simulink model "pv_array2"  (R2015a)
settings: Solver=ode45  StartTime=0.0  StopTime=10  RelTol=1e-3
undefined symbols (not defined in the file or in its folder): sigbuilder_block
libraries: powerlib x24
(part 2 of 2)

== system pv_array2/PV_array /PV module6/PV module/Photon Curr  ==
  "Tak " : Inport
  Trk : Inport  Port=2
  Isc,ref : Inport  Port=3
  "Insolation " : Inport  Port=4
  Ki : Inport  Port=5
  " " : Constant  Value=1000
  Divide : Product  Inputs=*/
  Product : Product
  Product1 : Product
  Sum1 : Sum  Inputs=|++
  Sum2 : Sum  Inputs=|+-
  "Iph " : Outport
  wires:
  "Tak "/1 -> Sum2/1
  Trk/1 -> Sum2/2
  Sum2/1 -> Product/2
  Product/1 -> Sum1/1
  Isc,ref/1 -> Sum1/2
  "Insolation "/1 -> Divide/1
  " "/1 -> Divide/2
  Divide/1 -> Product1/1
  Product1/1 -> "Iph "/1
  Sum1/1 -> Product1/2
  Ki/1 -> Product/1

== system pv_array2/PV_array /PV module6/PV module/Reverse Sat Cur  ==
  "Tak " : Inport
  "Isc ref " : Inport  Port=2
  q : Inport  Port=3
  Voc : Inport  Port=4
  k : Inport  Port=5
  "A " : Inport  Port=6
  "Constant " : Constant
  Divide : Product  Inputs=**////
  Fcn : Fcn  Expr=u(1)/(exp(u(2))-u(3))
  Mux : Mux  Inputs=3
  "Ns " : Constant  Value=36
  Irs : Outport
  wires:
  "Tak "/1 -> Divide/6
  "Ns "/1 -> Divide/4
  "Isc ref "/1 -> Mux/1
  Divide/1 -> Mux/2
  "Constant "/1 -> Mux/3
  Mux/1 -> Fcn/1
  Fcn/1 -> Irs/1
  q/1 -> Divide/1
  Voc/1 -> Divide/2
  k/1 -> Divide/3
  "A "/1 -> Divide/5

== system pv_array2/PV_array /PV module6/PV module/Sat Curr ==
  Irs : Inport
  Tak : Inport  Port=2
  Trk : Inport  Port=3
  q : Inport  Port=4
  Eg0 : Inport  Port=5
  k : Inport  Port=6
  B : Inport  Port=7
  " " : Constant
  Divide : Product  Inputs=*/
  Divide1 : Product  Inputs=***//
  Divide2 : Product  Inputs=*/
  Divide3 : Product  Inputs=*/
  Fcn : Fcn  Expr=(u(1))^3
  Math Function : Math  SaturateOnIntegerOverflow=on
  Product1 : Product  Inputs=3
  Sum : Sum  Inputs=|+-
  Is : Outport
  wires:
  Sum/1 -> Divide1/3
  Fcn/1 -> Product1/2
  Divide/1 -> Fcn/1
  Product1/1 -> Is/1
  Math Function/1 -> Product1/1
  Divide1/1 -> Math Function/1
  Tak/1 -> Divide3/2, Divide/1
  Irs/1 -> Product1/3
  " "/1 -> Divide3/1, Divide2/1
  Trk/1 -> Divide2/2, Divide/2
  Divide2/1 -> Sum/1
  Divide3/1 -> Sum/2
  q/1 -> Divide1/1
  Eg0/1 -> Divide1/2
  k/1 -> Divide1/4
  B/1 -> Divide1/5

== system pv_array2/PV_array /PV module7/PV module/Cel to Kel ==
  "Top " : Inport
  Add : Sum
  Add1 : Sum
  Cel to Kel : Constant  Value=273
  T(ref ^C)1 : Constant  Value=25
  "Tak " : Outport
  "Trk " : Outport  Port=2
  wires:
  Add/1 -> "Tak "/1
  Add1/1 -> "Trk "/1
  T(ref ^C)1/1 -> Add1/1
  Cel to Kel/1 -> Add1/2, Add/2
  "Top "/1 -> Add/1

== system pv_array2/PV_array /PV module7/PV module/NsAkt ==
  TaK : Inport
  Ns : Inport  Port=2
  k : Inport  Port=3
  A : Inport  Port=4
  Product : Product  Inputs=4
  Naskt : Outport
  wires:
  Product/1 -> Naskt/1
  TaK/1 -> Product/4
  Ns/1 -> Product/1
  k/1 -> Product/2
  A/1 -> Product/3

== system pv_array2/PV_array /PV module7/PV module/PV-Panel Current ==
  Is : Inport
  "Vpv " : Inport  Port=2
  NsAkT : Inport  Port=3
  "Iph " : Inport  Port=4
  Np : Inport  Port=5
  q : Inport  Port=6
  Fcn : Fcn  Expr=u(7)*u(2)-u(6)*u(2)*(exp((u(3)*(u(4)+u(5))/u(1)))-1)
  Mux : Mux  Inputs=7
  Rs : Gain  Gain=0.45
  Ipv : Outport
  wires:
  NsAkT/1 -> Mux/1
  Fcn/1 -> Ipv/1, Rs/1
  Rs/1 -> Mux/5
  "Iph "/1 -> Mux/7
  Is/1 -> Mux/6
  "Vpv "/1 -> Mux/4
  Mux/1 -> Fcn/1
  Np/1 -> Mux/2
  q/1 -> Mux/3

== system pv_array2/PV_array /PV module7/PV module/Photon Curr  ==
  "Tak " : Inport
  Trk : Inport  Port=2
  Isc,ref : Inport  Port=3
  "Insolation " : Inport  Port=4
  Ki : Inport  Port=5
  " " : Constant  Value=1000
  Divide : Product  Inputs=*/
  Product : Product
  Product1 : Product
  Sum1 : Sum  Inputs=|++
  Sum2 : Sum  Inputs=|+-
  "Iph " : Outport
  wires:
  "Tak "/1 -> Sum2/1
  Trk/1 -> Sum2/2
  Sum2/1 -> Product/2
  Product/1 -> Sum1/1
  Isc,ref/1 -> Sum1/2
  "Insolation "/1 -> Divide/1
  " "/1 -> Divide/2
  Divide/1 -> Product1/1
  Product1/1 -> "Iph "/1
  Sum1/1 -> Product1/2
  Ki/1 -> Product/1

== system pv_array2/PV_array /PV module7/PV module/Reverse Sat Cur  ==
  "Tak " : Inport
  "Isc ref " : Inport  Port=2
  q : Inport  Port=3
  Voc : Inport  Port=4
  k : Inport  Port=5
  "A " : Inport  Port=6
  "Constant " : Constant
  Divide : Product  Inputs=**////
  Fcn : Fcn  Expr=u(1)/(exp(u(2))-u(3))
  Mux : Mux  Inputs=3
  "Ns " : Constant  Value=36
  Irs : Outport
  wires:
  "Tak "/1 -> Divide/6
  "Ns "/1 -> Divide/4
  "Isc ref "/1 -> Mux/1
  Divide/1 -> Mux/2
  "Constant "/1 -> Mux/3
  Mux/1 -> Fcn/1
  Fcn/1 -> Irs/1
  q/1 -> Divide/1
  Voc/1 -> Divide/2
  k/1 -> Divide/3
  "A "/1 -> Divide/5

== system pv_array2/PV_array /PV module7/PV module/Sat Curr ==
  Irs : Inport
  Tak : Inport  Port=2
  Trk : Inport  Port=3
  q : Inport  Port=4
  Eg0 : Inport  Port=5
  k : Inport  Port=6
  B : Inport  Port=7
  " " : Constant
  Divide : Product  Inputs=*/
  Divide1 : Product  Inputs=***//
  Divide2 : Product  Inputs=*/
  Divide3 : Product  Inputs=*/
  Fcn : Fcn  Expr=(u(1))^3
  Math Function : Math  SaturateOnIntegerOverflow=on
  Product1 : Product  Inputs=3
  Sum : Sum  Inputs=|+-
  Is : Outport
  wires:
  Sum/1 -> Divide1/3
  Fcn/1 -> Product1/2
  Divide/1 -> Fcn/1
  Product1/1 -> Is/1
  Math Function/1 -> Product1/1
  Divide1/1 -> Math Function/1
  Tak/1 -> Divide3/2, Divide/1
  Irs/1 -> Product1/3
  " "/1 -> Divide3/1, Divide2/1
  Trk/1 -> Divide2/2, Divide/2
  Divide2/1 -> Sum/1
  Divide3/1 -> Sum/2
  q/1 -> Divide1/1
  Eg0/1 -> Divide1/2
  k/1 -> Divide1/4
  B/1 -> Divide1/5

== system pv_array2/PV_array /PV module8/PV module/Cel to Kel ==
  "Top " : Inport
  Add : Sum
  Add1 : Sum
  Cel to Kel : Constant  Value=273
  T(ref ^C)1 : Constant  Value=25
  "Tak " : Outport
  "Trk " : Outport  Port=2
  wires:
  Add/1 -> "Tak "/1
  Add1/1 -> "Trk "/1
  T(ref ^C)1/1 -> Add1/1
  Cel to Kel/1 -> Add1/2, Add/2
  "Top "/1 -> Add/1

== system pv_array2/PV_array /PV module8/PV module/NsAkt ==
  TaK : Inport
  Ns : Inport  Port=2
  k : Inport  Port=3
  A : Inport  Port=4
  Product : Product  Inputs=4
  Naskt : Outport
  wires:
  Product/1 -> Naskt/1
  TaK/1 -> Product/4
  Ns/1 -> Product/1
  k/1 -> Product/2
  A/1 -> Product/3

== system pv_array2/PV_array /PV module8/PV module/PV-Panel Current ==
  Is : Inport
  "Vpv " : Inport  Port=2
  NsAkT : Inport  Port=3
  "Iph " : Inport  Port=4
  Np : Inport  Port=5
  q : Inport  Port=6
  Fcn : Fcn  Expr=u(7)*u(2)-u(6)*u(2)*(exp((u(3)*(u(4)+u(5))/u(1)))-1)
  Mux : Mux  Inputs=7
  Rs : Gain  Gain=0.45
  Ipv : Outport
  wires:
  NsAkT/1 -> Mux/1
  Fcn/1 -> Ipv/1, Rs/1
  Rs/1 -> Mux/5
  "Iph "/1 -> Mux/7
  Is/1 -> Mux/6
  "Vpv "/1 -> Mux/4
  Mux/1 -> Fcn/1
  Np/1 -> Mux/2
  q/1 -> Mux/3

== system pv_array2/PV_array /PV module8/PV module/Photon Curr  ==
  "Tak " : Inport
  Trk : Inport  Port=2
  Isc,ref : Inport  Port=3
  "Insolation " : Inport  Port=4
  Ki : Inport  Port=5
  " " : Constant  Value=1000
  Divide : Product  Inputs=*/
  Product : Product
  Product1 : Product
  Sum1 : Sum  Inputs=|++
  Sum2 : Sum  Inputs=|+-
  "Iph " : Outport
  wires:
  "Tak "/1 -> Sum2/1
  Trk/1 -> Sum2/2
  Sum2/1 -> Product/2
  Product/1 -> Sum1/1
  Isc,ref/1 -> Sum1/2
  "Insolation "/1 -> Divide/1
  " "/1 -> Divide/2
  Divide/1 -> Product1/1
  Product1/1 -> "Iph "/1
  Sum1/1 -> Product1/2
  Ki/1 -> Product/1

== system pv_array2/PV_array /PV module8/PV module/Reverse Sat Cur  ==
  "Tak " : Inport
  "Isc ref " : Inport  Port=2
  q : Inport  Port=3
  Voc : Inport  Port=4
  k : Inport  Port=5
  "A " : Inport  Port=6
  "Constant " : Constant
  Divide : Product  Inputs=**////
  Fcn : Fcn  Expr=u(1)/(exp(u(2))-u(3))
  Mux : Mux  Inputs=3
  "Ns " : Constant  Value=36
  Irs : Outport
  wires:
  "Tak "/1 -> Divide/6
  "Ns "/1 -> Divide/4
  "Isc ref "/1 -> Mux/1
  Divide/1 -> Mux/2
  "Constant "/1 -> Mux/3
  Mux/1 -> Fcn/1
  Fcn/1 -> Irs/1
  q/1 -> Divide/1
  Voc/1 -> Divide/2
  k/1 -> Divide/3
  "A "/1 -> Divide/5

== system pv_array2/PV_array /PV module8/PV module/Sat Curr ==
  Irs : Inport
  Tak : Inport  Port=2
  Trk : Inport  Port=3
  q : Inport  Port=4
  Eg0 : Inport  Port=5
  k : Inport  Port=6
  B : Inport  Port=7
  " " : Constant
  Divide : Product  Inputs=*/
  Divide1 : Product  Inputs=***//
  Divide2 : Product  Inputs=*/
  Divide3 : Product  Inputs=*/
  Fcn : Fcn  Expr=(u(1))^3
  Math Function : Math  SaturateOnIntegerOverflow=on
  Product1 : Product  Inputs=3
  Sum : Sum  Inputs=|+-
  Is : Outport
  wires:
  Sum/1 -> Divide1/3
  Fcn/1 -> Product1/2
  Divide/1 -> Fcn/1
  Product1/1 -> Is/1
  Math Function/1 -> Product1/1
  Divide1/1 -> Math Function/1
  Tak/1 -> Divide3/2, Divide/1
  Irs/1 -> Product1/3
  " "/1 -> Divide3/1, Divide2/1
  Trk/1 -> Divide2/2, Divide/2
  Divide2/1 -> Sum/1
  Divide3/1 -> Sum/2
  q/1 -> Divide1/1
  Eg0/1 -> Divide1/2
  k/1 -> Divide1/4
  B/1 -> Divide1/5

== system pv_array2/PV_array /PV module9/PV module/Cel to Kel ==
  "Top " : Inport
  Add : Sum
  Add1 : Sum
  Cel to Kel : Constant  Value=273
  T(ref ^C)1 : Constant  Value=25
  "Tak " : Outport
  "Trk " : Outport  Port=2
  wires:
  Add/1 -> "Tak "/1
  Add1/1 -> "Trk "/1
  T(ref ^C)1/1 -> Add1/1
  Cel to Kel/1 -> Add1/2, Add/2
  "Top "/1 -> Add/1

== system pv_array2/PV_array /PV module9/PV module/NsAkt ==
  TaK : Inport
  Ns : Inport  Port=2
  k : Inport  Port=3
  A : Inport  Port=4
  Product : Product  Inputs=4
  Naskt : Outport
  wires:
  Product/1 -> Naskt/1
  TaK/1 -> Product/4
  Ns/1 -> Product/1
  k/1 -> Product/2
  A/1 -> Product/3

== system pv_array2/PV_array /PV module9/PV module/PV-Panel Current ==
  NsAkT : Inport
  Np : Inport  Port=2
  q : Inport  Port=3
  "Vpv " : Inport  Port=4
  Is : Inport  Port=5
  "Iph " : Inport  Port=6
  Display : Display
  Display1 : Display
  Display2 : Display
  Fcn : Fcn  Expr=u(7)*u(2)-u(6)*u(2)*(exp((u(3)*(u(4)+u(5))/u(1)))-1)
  Mux : Mux  Inputs=7
  Rs : Gain  Gain=0.45
  Ipv : Outport
  wires:
  NsAkT/1 -> Mux/1
  Fcn/1 -> Ipv/1, Display2/1, Rs/1
  "Iph "/1 -> Mux/6, Display/1
  Is/1 -> Mux/5, Display1/1
  "Vpv "/1 -> Mux/4
  Mux/1 -> Fcn/1
  Np/1 -> Mux/2
  q/1 -> Mux/3
  Rs/1 -> Mux/7

== system pv_array2/PV_array /PV module9/PV module/Photon Curr  ==
  "Tak " : Inport
  Trk : Inport  Port=2
  Isc,ref : Inport  Port=3
  "Insolation " : Inport  Port=4
  Ki : Inport  Port=5
  " " : Constant  Value=1000
  Divide : Product  Inputs=*/
  Product : Product
  Product1 : Product
  Sum1 : Sum  Inputs=|++
  Sum2 : Sum  Inputs=|+-
  "Iph " : Outport
  wires:
  "Tak "/1 -> Sum2/1
  Trk/1 -> Sum2/2
  Sum2/1 -> Product/2
  Product/1 -> Sum1/1
  Isc,ref/1 -> Sum1/2
  "Insolation "/1 -> Divide/1
  " "/1 -> Divide/2
  Divide/1 -> Product1/1
  Product1/1 -> "Iph "/1
  Sum1/1 -> Product1/2
  Ki/1 -> Product/1

== system pv_array2/PV_array /PV module9/PV module/Reverse Sat Cur  ==
  "Tak " : Inport
  "Isc ref " : Inport  Port=2
  q : Inport  Port=3
  Voc : Inport  Port=4
  k : Inport  Port=5
  "A " : Inport  Port=6
  "Constant " : Constant
  Divide : Product  Inputs=**////
  Fcn : Fcn  Expr=u(1)/(exp(u(2))-u(3))
  Mux : Mux  Inputs=3
  "Ns " : Constant  Value=36
  Irs : Outport
  wires:
  "Tak "/1 -> Divide/6
  "Ns "/1 -> Divide/4
  "Isc ref "/1 -> Mux/1
  Divide/1 -> Mux/2
  "Constant "/1 -> Mux/3
  Mux/1 -> Fcn/1
  Fcn/1 -> Irs/1
  q/1 -> Divide/1
  Voc/1 -> Divide/2
  k/1 -> Divide/3
  "A "/1 -> Divide/5

== system pv_array2/PV_array /PV module9/PV module/Sat Curr ==
  Irs : Inport
  Tak : Inport  Port=2
  Trk : Inport  Port=3
  q : Inport  Port=4
  Eg0 : Inport  Port=5
  k : Inport  Port=6
  B : Inport  Port=7
  " " : Constant
  Divide : Product  Inputs=*/
  Divide1 : Product  Inputs=***//
  Divide2 : Product  Inputs=*/
  Divide3 : Product  Inputs=*/
  Fcn : Fcn  Expr=(u(1))^3
  Math Function : Math  SaturateOnIntegerOverflow=on
  Product1 : Product  Inputs=3
  Sum : Sum  Inputs=|+-
  Is : Outport
  wires:
  Sum/1 -> Divide1/3
  Fcn/1 -> Product1/2
  Divide/1 -> Fcn/1
  Product1/1 -> Is/1
  Math Function/1 -> Product1/1
  Divide1/1 -> Math Function/1
  Tak/1 -> Divide3/2, Divide/1
  Irs/1 -> Product1/3
  " "/1 -> Divide3/1, Divide2/1
  Trk/1 -> Divide2/2, Divide/2
  Divide2/1 -> Sum/1
  Divide3/1 -> Sum/2
  q/1 -> Divide1/1
  Eg0/1 -> Divide1/2
  k/1 -> Divide1/4
  B/1 -> Divide1/5
